simulink library "BrickPi"  (R2018b)
settings: Solver=VariableStepAuto  StartTime=0.0  StopTime=10.0  RelTol=1e-3
libraries: raspberrypilib x50, hdlsllib x27, xpcutilitieslib x18, $bdroot x1
(part 2 of 4)

== system BrickPi/EV3_Infrared/Get_sensor_value ==
  SensorPort : Inport
  SensorType : Inport  Port=2
  Enable : EnablePort
  Merge2 : Merge  Inputs=3
  Subsystem : Subsystem
  Subsystem1 : Subsystem
  Subsystem2 : Subsystem
  Switch Case : SwitchCase  CaseConditions={1,2,3}
  Terminator : Terminator
  Proximity : Outport
  Heading : Outport  Port=2
  Distance : Outport  Port=3
  Remote : Outport  Port=4
  Error : Outport  Port=5
  wires:
  SensorType/1 -> Subsystem2/2(SensorType), Subsystem1/2(SensorType), Subsystem/2(SensorType), Switch Case/1
  Switch Case/4 -> Terminator/1
  Switch Case/1 -> Subsystem/Action
  Subsystem/1(Proximity) -> Proximity/1
  Subsystem/2(Error) -> Merge2/1
  Subsystem1/3(Error) -> Merge2/2
  Switch Case/2 -> Subsystem1/Action
  Merge2/1 -> Error/1
  Subsystem2/2(Error) -> Merge2/3
  Switch Case/3 -> Subsystem2/Action
  Subsystem1/1(Heading) -> Heading/1
  Subsystem1/2(Distance) -> Distance/1
  Subsystem2/1(Remote) -> Remote/1
  SensorPort/1 -> Subsystem/1(SensorPort), Subsystem1/1(SensorPort), Subsystem2/1(SensorPort)

== system BrickPi/EV3_Infrared/Set_sensor_type ==
  note: Check whether 4th element == 0xA5?
  note: Set sensor type
  SensorPort : Inport  OutDataTypeStr=uint8
  SensorType : Inport  Port=2
  Enable : EnablePort
  0xA5 : Constant  Value=165
  Add : Sum
  Address : Constant  VectorParams1D=off  OutDataTypeStr=uint8
  Constant2 : Constant  OutDataTypeStr=uint8
  Constant3 : Constant  OutDataTypeStr=uint8
  Mux1 : Mux
  NAND : Logic  Operator=NAND  IconShape=distinctive  AllPortsSameDT=off  OutDataTypeStr=boolean
  SPI Master Transfer1 : raspberrypilib/SPI Master Transfer  Priority=1  BoardProperty=Pi 3 Model B  SPIModule=uint32(0)  Mode=Master  BusSpeed=1000000  Pin=SPI0_CE1  FirstBitToTransfer=Most significant bit (MSB)  ClockMode=0  BlockFunction=Transfer  RegisterAddress=0  OutputDataType=int8  OutputDataLength=1
      settings: SourceProductName=Simulink Support Package for Raspberry Pi Hardware  SourceProductBaseCode=RASPPI
  SPI_MSG_SET_ SENSOR_TYPE : Constant  Value=12  OutMin=[1]  OutMax=[28]  OutDataTypeStr=uint8
  Selector1 : Selector  InputPortWidth=4  IndexOptions=Index vector (dialog)  Indices=[4]  OutputSizes=1
  Shift Arithmetic : ArithShift  BitShiftNumberSource=Input port  BitShiftNumber=8  BitShiftDirection=Left
      settings: InputPortMap=u0,p1
  Subtract : Sum  Inputs=+-
  Type Offset : Constant  Value=25  OutDataTypeStr=uint8
  Error : Outport
  wires:
  Mux1/1 -> SPI Master Transfer1/1
  SPI Master Transfer1/1 -> Selector1/1
  Address/1 -> Mux1/1
  SPI_MSG_SET_ SENSOR_TYPE/1 -> Mux1/2
  Selector1/1 -> NAND/1
  0xA5/1 -> NAND/2
  NAND/1 -> Error/1
  Subtract/1 -> Shift Arithmetic/2
  Constant3/1 -> Subtract/2
  SensorPort/1 -> Subtract/1
  Constant2/1 -> Shift Arithmetic/1
  Shift Arithmetic/1 -> Mux1/3
  SensorType/1 -> Add/1
  Type Offset/1 -> Add/2
  Add/1 -> Mux1/4

== system BrickPi/EV3_Ultrasonic/Get_sensor_value ==
  note: Which sensor type has been selected?
  SensorPort : Inport
  SensorType : Inport  Port=2  OutDataTypeStr=uint8
  Enable : EnablePort
  CM_INCHES : Subsystem
  LISTEN : Subsystem
  Merge1 : Merge
  Switch Case : SwitchCase  CaseConditions={[1,2],3}
  Terminator : Terminator
  cm : Outport
  inch : Outport  Port=2
  pres : Outport  Port=3
  Error : Outport  Port=4
  wires:
  SensorType/1 -> CM_INCHES/2(SensorType), Switch Case/1
  Switch Case/1 -> CM_INCHES/Action
  Switch Case/2 -> LISTEN/Action
  SensorPort/1 -> CM_INCHES/1(SensorPort), LISTEN/1(SensorPort)
  CM_INCHES/1(cm) -> cm/1
  Merge1/1 -> Error/1
  CM_INCHES/3(Error) -> Merge1/1
  LISTEN/2(Error) -> Merge1/2
  LISTEN/1(presence) -> pres/1
  CM_INCHES/2(inch) -> inch/1
  Switch Case/3 -> Terminator/1

== system BrickPi/EV3_Ultrasonic/Set_sensor_type ==
  note: Set sensor type
  note: Check whether 4th element == 0xA5?
  SensorPort : Inport  OutDataTypeStr=uint8
  SensorType : Inport  Port=2  OutDataTypeStr=uint8
  Enable : EnablePort
  0xA5 : Constant  Value=165
  Address : Constant  VectorParams1D=off  OutDataTypeStr=uint8
  Constant2 : Constant  OutDataTypeStr=uint8
  Constant3 : Constant  OutDataTypeStr=uint8
  Mux1 : Mux
  NAND : Logic  Operator=NAND  IconShape=distinctive  AllPortsSameDT=off  OutDataTypeStr=boolean
  SPI Master Transfer1 : raspberrypilib/SPI Master Transfer  Priority=1  BoardProperty=Pi 3 Model B  SPIModule=uint32(0)  Mode=Master  BusSpeed=1000000  Pin=SPI0_CE1  FirstBitToTransfer=Most significant bit (MSB)  ClockMode=0  BlockFunction=Transfer  RegisterAddress=0  OutputDataType=int8  OutputDataLength=1
      settings: SourceProductName=Simulink Support Package for Raspberry Pi Hardware  SourceProductBaseCode=RASPPI
  SPI_MSG_SET_ SENSOR_TYPE : Constant  Value=12  OutMin=[1]  OutMax=[28]  OutDataTypeStr=uint8
  Selector1 : Selector  InputPortWidth=4  IndexOptions=Index vector (dialog)  Indices=[4]  OutputSizes=1
  Sensor type offset : Constant  Value=22  OutDataTypeStr=uint8
  Shift Arithmetic : ArithShift  BitShiftNumberSource=Input port  BitShiftNumber=8  BitShiftDirection=Left
      settings: InputPortMap=u0,p1
  Subtract : Sum  Inputs=+-
  Sum : Sum
  Error : Outport  InitialOutput=[1]
  wires:
  Sensor type offset/1 -> Sum/2
  SensorType/1 -> Sum/1
  Sum/1 -> Mux1/4
  Shift Arithmetic/1 -> Mux1/3
  Constant2/1 -> Shift Arithmetic/1
  SensorPort/1 -> Subtract/1
  Constant3/1 -> Subtract/2
  Subtract/1 -> Shift Arithmetic/2
  NAND/1 -> Error/1
  0xA5/1 -> NAND/2
  Selector1/1 -> NAND/1
  SPI_MSG_SET_ SENSOR_TYPE/1 -> Mux1/2
  Address/1 -> Mux1/1
  SPI Master Transfer1/1 -> Selector1/1
  Mux1/1 -> SPI Master Transfer1/1

== system BrickPi/Motor_Encoder/Get Encoder Value ==
  note: Use only when "Reset on external signal" selected
  note: Get motor encoder
  MotorPort : Inport
  ResetMode : Inport  Port=2
  ExtSignal : Inport  Port=3
  Enable : EnablePort
  0xA5 : Constant  Value=165
  "Address " : Constant  OutDataTypeStr=uint8
  Address3 : Constant  Value=[0 0 0 0 0 0 0 0]  OutDataTypeStr=uint8
  "Byte Packing " : xpcutilitieslib/Byte Packing   MaskPackedDataType=int32  MaskUnpackedDataTypes={'uint8', 'uint8', 'uint8', 'uint8'}  MaskAlignment=1
  Bytes[3-7] : Selector  IndexMode=Zero-based  InputPortWidth=10  IndexOptions=Index vector (dialog)  Indices=[3 4 5 6 7]  OutputSizes=1
  Demux : Demux  Outputs=5
  Mux2 : Mux  Inputs=3
  NAND : Logic  Operator=NAND  IconShape=distinctive  AllPortsSameDT=off  OutDataTypeStr=boolean
  SPI Master Transfer2 : raspberrypilib/SPI Master Transfer  Priority=6  BoardProperty=Pi 3 Model B  SPIModule=uint32(0)  Mode=Master  BusSpeed=1000000  Pin=SPI0_CE1  FirstBitToTransfer=Most significant bit (MSB)  ClockMode=0  BlockFunction=Transfer  RegisterAddress=0  OutputDataType=int8  OutputDataLength=1
      settings: SourceProductName=Simulink Support Package for Raspberry Pi Hardware  SourceProductBaseCode=RASPPI
  SPI_MSG_GET_ MOTOR_ENCODER offset : Constant  Value=29  OutDataTypeStr=uint8
  Sum : Sum  OutDataTypeStr=uint8
  Switch Case : SwitchCase
  Switch Case Action Subsystem : Subsystem  TreatAsAtomicUnit=on
  Terminator : Terminator
  Value : Outport
  Error : Outport  Port=2
  wires:
  SPI_MSG_GET_ MOTOR_ENCODER offset/1 -> Sum/2
  SPI Master Transfer2/1 -> Bytes[3-7]/1
  Bytes[3-7]/1 -> Demux/1
  "Byte Packing "/1 -> Value/1
  Demux/2 -> "Byte Packing "/4
  0xA5/1 -> NAND/1
  Demux/1 -> NAND/2
  Demux/3 -> "Byte Packing "/3
  Demux/4 -> "Byte Packing "/2
  "Address "/1 -> Mux2/1
  Demux/5 -> "Byte Packing "/1
  MotorPort/1 -> Switch Case Action Subsystem/2(MotorPort), Sum/1
  Mux2/1 -> SPI Master Transfer2/1
  Sum/1 -> Mux2/2
  NAND/1 -> Error/1
  Address3/1 -> Mux2/3
  ResetMode/1 -> Switch Case/1
  Switch Case/2 -> Terminator/1
  Switch Case/1 -> Switch Case Action Subsystem/Action
  ExtSignal/1 -> Switch Case Action Subsystem/1(ExtSignal)

== system BrickPi/Motor_Encoder/Reset Encoder once ==
  MotorPort : Inport
  Enable : EnablePort
  Encoder : Subsystem  AncestorBlock=BrickPi/Motor_Encoder/Subsystem
  Motor_Offset : Subsystem
  Error : Outport
  wires:
  Encoder/1(Value) -> Motor_Offset/1(Offset)
  MotorPort/1 -> Motor_Offset/2(MotorPort), Encoder/1(MotorPort)
  Encoder/2(Error) -> Error/1

== system BrickPi/Motor_Offset/If Action Subsystem ==
  note: Set offset value
  Offset : Inport
  Action Port : ActionPort  ActionType=then
  "Address " : Constant  OutDataTypeStr=uint8
  Bit Shift : hdlsllib/Logic and Bit Operations/Bit Shift  mode=Shift Right Logical  N=24
      settings: SourceProductName=HDL Coder  SourceProductBaseCode=HD
  Bit Shift1 : hdlsllib/Logic and Bit Operations/Bit Shift  mode=Shift Right Logical  N=16
      settings: SourceProductName=HDL Coder  SourceProductBaseCode=HD
  Bit Shift2 : hdlsllib/Logic and Bit Operations/Bit Shift  mode=Shift Right Logical  N=8
      settings: SourceProductName=HDL Coder  SourceProductBaseCode=HD
  "Byte Unpacking " : xpcutilitieslib/Byte Unpacking   MaskUnpackedDataTypes={'uint8'}  MaskUnpackedDataSizes={[1]}  MaskAlignment=1
      settings: SourceProductName=Simulink Real-Time  SourceProductBaseCode=XP
  Constant2 : Constant  OutDataTypeStr=uint8
  Constant3 : Constant  OutDataTypeStr=uint8
  Data Type Conversion{,1..3} (4 alike) : DataTypeConversion  OutDataTypeStr=uint8
  MotorPort : Constant  Value=MotorPort  OutDataTypeStr=uint8
  Mux2 : Mux  Inputs=7
  SPI Master Transfer2 : raspberrypilib/SPI Master Transfer  Priority=6  BoardProperty=Pi 3 Model B  SPIModule=uint32(0)  Mode=Master  BusSpeed=1000000  Pin=SPI0_CE1  FirstBitToTransfer=Most significant bit (MSB)  ClockMode=0  BlockFunction=Transfer  RegisterAddress=0  OutputDataType=int8  OutputDataLength=1
      settings: SourceProductName=Simulink Support Package for Raspberry Pi Hardware  SourceProductBaseCode=RASPPI
  SPI_MSG_ OFFSET_ENCODER : Constant  Value=29  OutMin=[1]  OutDataTypeStr=uint8
  Shift Arithmetic : ArithShift  BitShiftNumberSource=Input port  BitShiftNumber=8  BitShiftDirection=Left
      settings: InputPortMap=u0,p1
  Subtract : Sum  Inputs=+-
  Terminator : Terminator
  wires:
  Data Type Conversion2/1 -> Mux2/6
  Constant2/1 -> Shift Arithmetic/1
  Data Type Conversion/1 -> Mux2/4
  Data Type Conversion3/1 -> Mux2/7
  MotorPort/1 -> Subtract/1
  SPI_MSG_ OFFSET_ENCODER/1 -> Mux2/2
  Subtract/1 -> Shift Arithmetic/2
  SPI Master Transfer2/1 -> Terminator/1
  Data Type Conversion1/1 -> Mux2/5
  "Address "/1 -> Mux2/1
  Bit Shift1/1 -> Data Type Conversion1/1
  Constant3/1 -> Subtract/2
  Bit Shift/1 -> Data Type Conversion/1
  Mux2/1 -> SPI Master Transfer2/1
  Shift Arithmetic/1 -> Mux2/3
  Bit Shift2/1 -> Data Type Conversion2/1
  Offset/1 -> Bit Shift1/1, Bit Shift2/1, Data Type Conversion3/1, Bit Shift/1

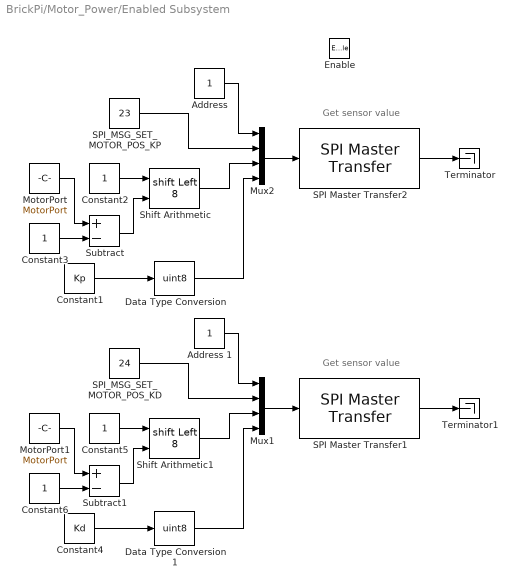
== system BrickPi/Motor_Power/Enabled Subsystem ==
  note: Get sensor value
  note: Get sensor value
  Enable : EnablePort
  "Address " : Constant  OutDataTypeStr=uint8
  Address 1 : Constant  OutDataTypeStr=uint8
  Constant1 : Constant  Value=Kp
  Constant{2..3,5..6} (4 alike) : Constant  OutDataTypeStr=uint8
  Constant4 : Constant  Value=Kd
  Data Type Conversion : DataTypeConversion  OutDataTypeStr=uint8
  Data Type Conversion1 : DataTypeConversion  OutDataTypeStr=uint8
  MotorPort : Constant  Value=MotorPort  OutDataTypeStr=uint8
  MotorPort1 : Constant  Value=MotorPort  OutDataTypeStr=uint8
  Mux1 : Mux
  Mux2 : Mux
  SPI Master Transfer1 : raspberrypilib/SPI Master Transfer  Priority=6  BoardProperty=Pi 3 Model B  SPIModule=uint32(0)  Mode=Master  BusSpeed=1000000  Pin=SPI0_CE1  FirstBitToTransfer=Most significant bit (MSB)  ClockMode=0  BlockFunction=Transfer  RegisterAddress=0  OutputDataType=int8  OutputDataLength=1
      settings: SourceProductName=Simulink Support Package for Raspberry Pi Hardware  SourceProductBaseCode=RASPPI
  SPI Master Transfer2 : raspberrypilib/SPI Master Transfer  Priority=6  BoardProperty=Pi 3 Model B  SPIModule=uint32(0)  Mode=Master  BusSpeed=1000000  Pin=SPI0_CE1  FirstBitToTransfer=Most significant bit (MSB)  ClockMode=0  BlockFunction=Transfer  RegisterAddress=0  OutputDataType=int8  OutputDataLength=1
      settings: SourceProductName=Simulink Support Package for Raspberry Pi Hardware  SourceProductBaseCode=RASPPI
  SPI_MSG_SET_ MOTOR_POS_KD : Constant  Value=24  OutMin=[1]  OutMax=[28]  OutDataTypeStr=uint8
  SPI_MSG_SET_ MOTOR_POS_KP : Constant  Value=23  OutMin=[1]  OutMax=[28]  OutDataTypeStr=uint8
  Shift Arithmetic : ArithShift  BitShiftNumberSource=Input port  BitShiftNumber=8  BitShiftDirection=Left
      settings: InputPortMap=u0,p1
  Shift Arithmetic1 : ArithShift  BitShiftNumberSource=Input port  BitShiftNumber=8  BitShiftDirection=Left
      settings: InputPortMap=u0,p1
  Subtract : Sum  Inputs=+-
  Subtract1 : Sum  Inputs=+-
  Terminator : Terminator
  Terminator1 : Terminator
  wires:
  SPI_MSG_SET_ MOTOR_POS_KP/1 -> Mux2/2
  Constant3/1 -> Subtract/2
  SPI Master Transfer2/1 -> Terminator/1
  Constant1/1 -> Data Type Conversion/1
  Data Type Conversion/1 -> Mux2/4
  MotorPort/1 -> Subtract/1
  Shift Arithmetic/1 -> Mux2/3
  "Address "/1 -> Mux2/1
  Constant2/1 -> Shift Arithmetic/1
  Mux2/1 -> SPI Master Transfer2/1
  Subtract/1 -> Shift Arithmetic/2
  Subtract1/1 -> Shift Arithmetic1/2
  Constant5/1 -> Shift Arithmetic1/1
  MotorPort1/1 -> Subtract1/1
  Mux1/1 -> SPI Master Transfer1/1
  Address 1/1 -> Mux1/1
  Shift Arithmetic1/1 -> Mux1/3
  Constant6/1 -> Subtract1/2
  Data Type Conversion1/1 -> Mux1/4
  SPI Master Transfer1/1 -> Terminator1/1
  SPI_MSG_SET_ MOTOR_POS_KD/1 -> Mux1/2
  Constant4/1 -> Data Type Conversion1/1

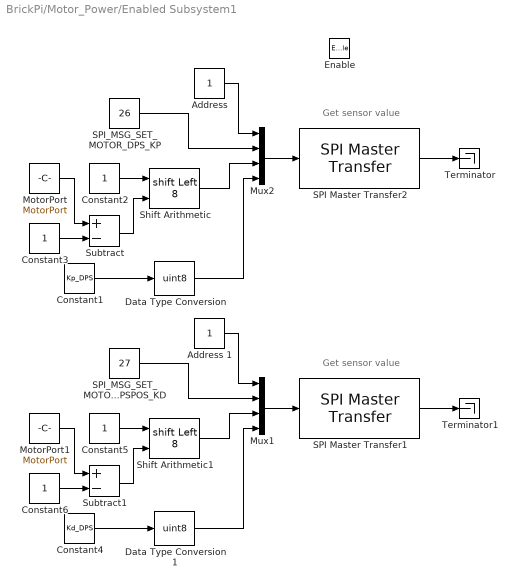
== system BrickPi/Motor_Power/Enabled Subsystem1 ==
  note: Get sensor value
  note: Get sensor value
  Enable : EnablePort
  "Address " : Constant  OutDataTypeStr=uint8
  Address 1 : Constant  OutDataTypeStr=uint8
  Constant1 : Constant  Value=Kp_DPS
  Constant{2..3,5..6} (4 alike) : Constant  OutDataTypeStr=uint8
  Constant4 : Constant  Value=Kd_DPS
  Data Type Conversion : DataTypeConversion  OutDataTypeStr=uint8
  Data Type Conversion1 : DataTypeConversion  OutDataTypeStr=uint8
  MotorPort : Constant  Value=MotorPort  OutDataTypeStr=uint8
  MotorPort1 : Constant  Value=MotorPort  OutDataTypeStr=uint8
  Mux1 : Mux
  Mux2 : Mux
  SPI Master Transfer1 : raspberrypilib/SPI Master Transfer  Priority=6  BoardProperty=Pi 3 Model B  SPIModule=uint32(0)  Mode=Master  BusSpeed=1000000  Pin=SPI0_CE1  FirstBitToTransfer=Most significant bit (MSB)  ClockMode=0  BlockFunction=Transfer  RegisterAddress=0  OutputDataType=int8  OutputDataLength=1
      settings: SourceProductName=Simulink Support Package for Raspberry Pi Hardware  SourceProductBaseCode=RASPPI
  SPI Master Transfer2 : raspberrypilib/SPI Master Transfer  Priority=6  BoardProperty=Pi 3 Model B  SPIModule=uint32(0)  Mode=Master  BusSpeed=1000000  Pin=SPI0_CE1  FirstBitToTransfer=Most significant bit (MSB)  ClockMode=0  BlockFunction=Transfer  RegisterAddress=0  OutputDataType=int8  OutputDataLength=1
      settings: SourceProductName=Simulink Support Package for Raspberry Pi Hardware  SourceProductBaseCode=RASPPI
  SPI_MSG_SET_ MOTOR_DPSPOS_KD : Constant  Value=27  OutMin=[1]  OutMax=[28]  OutDataTypeStr=uint8
  SPI_MSG_SET_ MOTOR_DPS_KP : Constant  Value=26  OutMin=[1]  OutMax=[28]  OutDataTypeStr=uint8
  Shift Arithmetic : ArithShift  BitShiftNumberSource=Input port  BitShiftNumber=8  BitShiftDirection=Left
      settings: InputPortMap=u0,p1
  Shift Arithmetic1 : ArithShift  BitShiftNumberSource=Input port  BitShiftNumber=8  BitShiftDirection=Left
      settings: InputPortMap=u0,p1
  Subtract : Sum  Inputs=+-
  Subtract1 : Sum  Inputs=+-
  Terminator : Terminator
  Terminator1 : Terminator
  wires:
  SPI_MSG_SET_ MOTOR_DPS_KP/1 -> Mux2/2
  Constant3/1 -> Subtract/2
  SPI Master Transfer2/1 -> Terminator/1
  Constant1/1 -> Data Type Conversion/1
  Data Type Conversion/1 -> Mux2/4
  MotorPort/1 -> Subtract/1
  Shift Arithmetic/1 -> Mux2/3
  "Address "/1 -> Mux2/1
  Constant2/1 -> Shift Arithmetic/1
  Mux2/1 -> SPI Master Transfer2/1
  Subtract/1 -> Shift Arithmetic/2
  Subtract1/1 -> Shift Arithmetic1/2
  Constant5/1 -> Shift Arithmetic1/1
  MotorPort1/1 -> Subtract1/1
  Mux1/1 -> SPI Master Transfer1/1
  Address 1/1 -> Mux1/1
  Shift Arithmetic1/1 -> Mux1/3
  Constant6/1 -> Subtract1/2
  Data Type Conversion1/1 -> Mux1/4
  SPI Master Transfer1/1 -> Terminator1/1
  SPI_MSG_SET_ MOTOR_DPSPOS_KD/1 -> Mux1/2
  Constant4/1 -> Data Type Conversion1/1

== system BrickPi/Motor_Power/Subsystem ==
  Choice : Inport
  Power : Inport  Port=2
  Position : Inport  Port=3
  DPS : Inport  Port=4
  Action Port : ActionPort  ActionType=then
  Set_DPS : Subsystem
  Set_Limit : Subsystem
  Set_Position : Subsystem
  Set_Power : Subsystem
  Switch Case : SwitchCase  CaseConditions={1,2,3,4}
  Terminator : Terminator
  wires:
  Switch Case/3 -> Set_DPS/Action
  DPS/1 -> Set_DPS/1(DPS), Set_Limit/2(DPS)
  Switch Case/1 -> Set_Power/Action
  Power/1 -> Set_Power/1(Power), Set_Limit/1(Power)
  Choice/1 -> Switch Case/1
  Switch Case/5 -> Terminator/1
  Position/1 -> Set_Position/1(Position)
  Switch Case/2 -> Set_Position/Action
  Switch Case/4 -> Set_Limit/Action

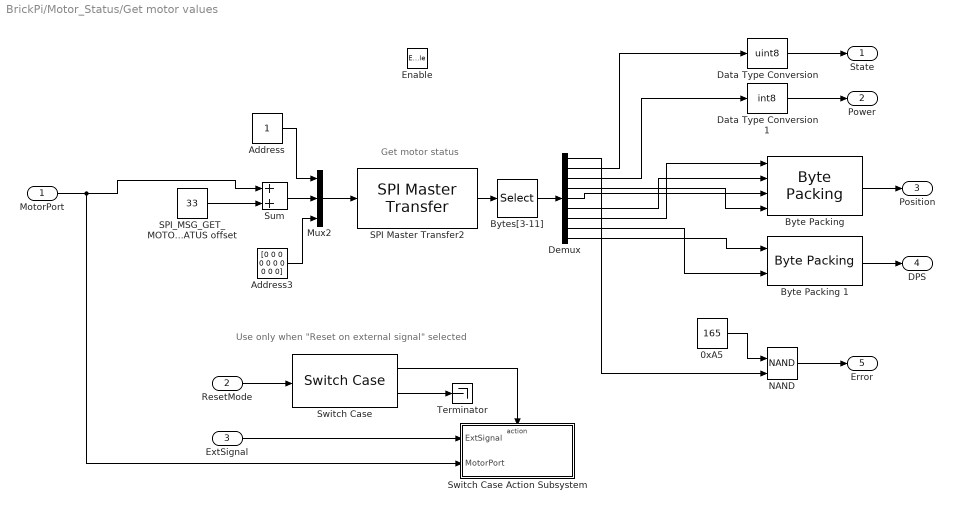
== system BrickPi/Motor_Status/Get motor values ==
  note: Get motor status
  note: Use only when "Reset on external signal" selected
  MotorPort : Inport
  ResetMode : Inport  Port=2
  ExtSignal : Inport  Port=3
  Enable : EnablePort
  0xA5 : Constant  Value=165
  "Address " : Constant  OutDataTypeStr=uint8
  Address3 : Constant  Value=[0 0 0 0 0 0 0 0 0 0]  OutDataTypeStr=uint8
  "Byte Packing " : xpcutilitieslib/Byte Packing   MaskPackedDataType=int32  MaskUnpackedDataTypes={'uint8', 'uint8', 'uint8', 'uint8'}  MaskAlignment=1
  Byte Packing 1 : xpcutilitieslib/Byte Packing   MaskPackedDataType=int16  MaskUnpackedDataTypes={'uint8','uint8'}  MaskAlignment=1
  Bytes[3-11] : Selector  IndexMode=Zero-based  InputPortWidth=12  IndexOptions=Index vector (dialog)  Indices=[3 4 5 6 7 8 9 10 11]  OutputSizes=1
  Data Type Conversion : DataTypeConversion  OutDataTypeStr=uint8
  Data Type Conversion1 : DataTypeConversion  OutDataTypeStr=int8
  Demux : Demux  Outputs=9
  Mux2 : Mux  Inputs=3
  NAND : Logic  Operator=NAND  IconShape=distinctive  AllPortsSameDT=off  OutDataTypeStr=boolean
  SPI Master Transfer2 : raspberrypilib/SPI Master Transfer  Priority=6  BoardProperty=Pi 3 Model B  SPIModule=uint32(0)  Mode=Master  BusSpeed=1000000  Pin=SPI0_CE1  FirstBitToTransfer=Most significant bit (MSB)  ClockMode=0  BlockFunction=Transfer  RegisterAddress=0  OutputDataType=int8  OutputDataLength=1
      settings: SourceProductName=Simulink Support Package for Raspberry Pi Hardware  SourceProductBaseCode=RASPPI
  SPI_MSG_GET_ MOTOR_STATUS offset : Constant  Value=33  OutMin=[1]  OutDataTypeStr=uint8
  Sum : Sum  OutDataTypeStr=uint8
  Switch Case : SwitchCase
  Switch Case Action Subsystem : Subsystem  TreatAsAtomicUnit=on
  Terminator : Terminator
  State : Outport
  Power : Outport  Port=2
  Position : Outport  Port=3
  DPS : Outport  Port=4
  Error : Outport  Port=5
  wires:
  Demux/2 -> Data Type Conversion/1
  Mux2/1 -> SPI Master Transfer2/1
  "Address "/1 -> Mux2/1
  Demux/9 -> Byte Packing 1/1
  Demux/1 -> NAND/2
  Demux/7 -> "Byte Packing "/1
  Demux/6 -> "Byte Packing "/2
  Bytes[3-11]/1 -> Demux/1
  SPI Master Transfer2/1 -> Bytes[3-11]/1
  Demux/8 -> Byte Packing 1/2
  SPI_MSG_GET_ MOTOR_STATUS offset/1 -> Sum/2
  Sum/1 -> Mux2/2
  MotorPort/1 -> Switch Case Action Subsystem/2(MotorPort), Sum/1
  0xA5/1 -> NAND/1
  Demux/3 -> Data Type Conversion1/1
  Address3/1 -> Mux2/3
  Demux/5 -> "Byte Packing "/3
  Demux/4 -> "Byte Packing "/4
  Byte Packing 1/1 -> DPS/1
  "Byte Packing "/1 -> Position/1
  NAND/1 -> Error/1
  Data Type Conversion1/1 -> Power/1
  Data Type Conversion/1 -> State/1
  ExtSignal/1 -> Switch Case Action Subsystem/1(ExtSignal)
  ResetMode/1 -> Switch Case/1
  Switch Case/1 -> Switch Case Action Subsystem/Action
  Switch Case/2 -> Terminator/1

== system BrickPi/Motor_Status/Reset Encoder once ==
  MotorPort : Inport
  Enable : EnablePort
  Encoder : Subsystem  AncestorBlock=BrickPi/Motor_Encoder/Subsystem
  Motor_Offset : Subsystem
  Error : Outport
  wires:
  Encoder/1(Value) -> Motor_Offset/1(Offset)
  MotorPort/1 -> Motor_Offset/2(MotorPort), Encoder/1(MotorPort)
  Encoder/2(Error) -> Error/1

== system BrickPi/NXT_Color/Get_sensor_value ==
  note: Which sensor type has been selected?
  SensorPort : Inport
  SensorType : Inport  Port=2  OutDataTypeStr=uint8
  Enable : EnablePort
  FULL : Subsystem
  Merge : Merge
  Merge1 : Merge
  R_G_B_OFF : Subsystem
  Switch Case : SwitchCase  CaseConditions={[1,2,3,5],4}
  Terminator : Terminator
  Values : Outport
  Error : Outport  Port=2
  wires:
  Switch Case/1 -> R_G_B_OFF/Action
  SensorType/1 -> R_G_B_OFF/2(SensorType), Switch Case/1
  Switch Case/2 -> FULL/Action
  SensorPort/1 -> R_G_B_OFF/1(SensorPort), FULL/1(SensorPort)
  Merge/1 -> Error/1
  FULL/2(Error) -> Merge/2
  R_G_B_OFF/2(Error) -> Merge/1
  Merge1/1 -> Values/1
  R_G_B_OFF/1(Value) -> Merge1/1
  FULL/1(Value) -> Merge1/2
  Switch Case/3 -> Terminator/1

== system BrickPi/NXT_Color/Set_sensor_type ==
  note: Set sensor type
  note: Check whether 4th element == 0xA5?
  SensorPort : Inport  OutDataTypeStr=uint8
  SensorType : Inport  Port=2  OutDataTypeStr=uint8
  Enable : EnablePort
  0xA5 : Constant  Value=165
  Address : Constant  VectorParams1D=off  OutDataTypeStr=uint8
  Constant2 : Constant  OutDataTypeStr=uint8
  Constant3 : Constant  OutDataTypeStr=uint8
  Mux1 : Mux
  NAND : Logic  Operator=NAND  IconShape=distinctive  AllPortsSameDT=off  OutDataTypeStr=boolean
  SPI Master Transfer1 : raspberrypilib/SPI Master Transfer  Priority=1  BoardProperty=Pi 3 Model B  SPIModule=uint32(0)  Mode=Master  BusSpeed=1000000  Pin=SPI0_CE1  FirstBitToTransfer=Most significant bit (MSB)  ClockMode=0  BlockFunction=Transfer  RegisterAddress=0  OutputDataType=int8  OutputDataLength=1
      settings: SourceProductName=Simulink Support Package for Raspberry Pi Hardware  SourceProductBaseCode=RASPPI
  SPI_MSG_SET_ SENSOR_TYPE : Constant  Value=12  OutMin=[1]  OutMax=[28]  OutDataTypeStr=uint8
  Selector1 : Selector  InputPortWidth=4  IndexOptions=Index vector (dialog)  Indices=[4]  OutputSizes=1
  Sensor type offset : Constant  Value=8  OutDataTypeStr=uint8
  Shift Arithmetic : ArithShift  BitShiftNumberSource=Input port  BitShiftNumber=8  BitShiftDirection=Left
      settings: InputPortMap=u0,p1
  Subtract : Sum  Inputs=+-
  Sum : Sum
  Error : Outport
  wires:
  Sensor type offset/1 -> Sum/2
  SensorType/1 -> Sum/1
  Sum/1 -> Mux1/4
  Shift Arithmetic/1 -> Mux1/3
  Constant2/1 -> Shift Arithmetic/1
  SensorPort/1 -> Subtract/1
  Constant3/1 -> Subtract/2
  Subtract/1 -> Shift Arithmetic/2
  NAND/1 -> Error/1
  0xA5/1 -> NAND/2
  Selector1/1 -> NAND/1
  SPI_MSG_SET_ SENSOR_TYPE/1 -> Mux1/2
  Address/1 -> Mux1/1
  SPI Master Transfer1/1 -> Selector1/1
  Mux1/1 -> SPI Master Transfer1/1

== system BrickPi/NXT_Light/Get_sensor_value ==
  note: Get sensor value
  SensorPort : Inport
  SensorType : Inport  Port=2  OutDataTypeStr=uint8
  Enable : EnablePort
  0xA5 : Constant  Value=165
  "Address " : Constant  OutDataTypeStr=uint8
  Address3 : Constant  Value=[0 0 0 0 0 0]  OutDataTypeStr=uint8
  "Byte Packing " : xpcutilitieslib/Byte Packing   MaskPackedDataType=uint16  MaskUnpackedDataTypes={'uint8', 'uint8'}  MaskAlignment=1
  Bytes[3-7] : Selector  IndexMode=Zero-based  InputPortWidth=8  IndexOptions=Index vector (dialog)  Indices=[3 4 5 6 7]  OutputSizes=1
  Demux : Demux  Outputs=5
  Equal : RelationalOperator  Operator=~=  OutDataTypeStr=boolean  RndMeth=Simplest
  Equal1 : RelationalOperator  Operator=~=  OutDataTypeStr=boolean  RndMeth=Simplest
  Equal2 : RelationalOperator  Operator=~=  OutDataTypeStr=boolean  RndMeth=Simplest
  Mux : Mux  Inputs=3
  Mux2 : Mux  Inputs=3
  SPI Master Transfer2 : raspberrypilib/SPI Master Transfer  Priority=6  BoardProperty=Pi 3 Model B  SPIModule=uint32(0)  Mode=Master  BusSpeed=1000000  Pin=SPI0_CE1  FirstBitToTransfer=Most significant bit (MSB)  ClockMode=0  BlockFunction=Transfer  RegisterAddress=0  OutputDataType=int8  OutputDataLength=1
      settings: SourceProductName=Simulink Support Package for Raspberry Pi Hardware  SourceProductBaseCode=RASPPI
  SPI_MSG_GET_ SENSOR offset : Constant  Value=12  OutMin=[1]  OutMax=[28]  OutDataTypeStr=uint8
  Sensor type offset : Constant  Value=6  OutDataTypeStr=uint8
  Sum : Sum  OutDataTypeStr=uint8
  Sum1 : Sum
  Valid data : Constant  Value=0  OutDataTypeStr=uint8
  Value : Outport
  Error : Outport  Port=2
  wires:
  Sensor type offset/1 -> Sum1/2
  SensorType/1 -> Sum1/1
  Sum1/1 -> Equal/1
  Equal2/1 -> Mux/1
  Demux/1 -> Equal2/2
  Equal1/1 -> Mux/3
  Mux/1 -> Error/1
  Equal/1 -> Mux/2
  Demux/3 -> Equal1/1
  Valid data/1 -> Equal1/2
  0xA5/1 -> Equal2/1
  Demux/2 -> Equal/2
  Bytes[3-7]/1 -> Demux/1
  SensorPort/1 -> Sum/1
  SPI_MSG_GET_ SENSOR offset/1 -> Sum/2
  Sum/1 -> Mux2/2
  "Address "/1 -> Mux2/1
  Mux2/1 -> SPI Master Transfer2/1
  SPI Master Transfer2/1 -> Bytes[3-7]/1
  Address3/1 -> Mux2/3
  "Byte Packing "/1 -> Value/1
  Demux/4 -> "Byte Packing "/2
  Demux/5 -> "Byte Packing "/1

== system BrickPi/NXT_Light/Set_sensor_type ==
  note: Set sensor type
  note: Check whether 4th element == 0xA5?
  SensorPort : Inport  OutDataTypeStr=uint8
  SensorType : Inport  Port=2  OutDataTypeStr=uint8
  Enable : EnablePort
  0xA5 : Constant  Value=165
  Address : Constant  VectorParams1D=off  OutDataTypeStr=uint8
  Constant2 : Constant  OutDataTypeStr=uint8
  Constant3 : Constant  OutDataTypeStr=uint8
  Mux1 : Mux
  NAND : Logic  Operator=NAND  IconShape=distinctive  AllPortsSameDT=off  OutDataTypeStr=boolean
  SPI Master Transfer1 : raspberrypilib/SPI Master Transfer  Priority=1  BoardProperty=Pi 3 Model B  SPIModule=uint32(0)  Mode=Master  BusSpeed=1000000  Pin=SPI0_CE1  FirstBitToTransfer=Most significant bit (MSB)  ClockMode=0  BlockFunction=Transfer  RegisterAddress=0  OutputDataType=int8  OutputDataLength=1
      settings: SourceProductName=Simulink Support Package for Raspberry Pi Hardware  SourceProductBaseCode=RASPPI
  SPI_MSG_SET_ SENSOR_TYPE : Constant  Value=12  OutMin=[1]  OutMax=[28]  OutDataTypeStr=uint8
  Selector1 : Selector  InputPortWidth=4  IndexOptions=Index vector (dialog)  Indices=[4]  OutputSizes=1
  Sensor type offset : Constant  Value=6  OutDataTypeStr=uint8
  Shift Arithmetic : ArithShift  BitShiftNumberSource=Input port  BitShiftNumber=8  BitShiftDirection=Left
      settings: InputPortMap=u0,p1
  Subtract : Sum  Inputs=+-
  Sum : Sum
  Error : Outport
  wires:
  Sensor type offset/1 -> Sum/2
  SensorType/1 -> Sum/1
  Sum/1 -> Mux1/4
  Shift Arithmetic/1 -> Mux1/3
  Constant2/1 -> Shift Arithmetic/1
  SensorPort/1 -> Subtract/1
  Constant3/1 -> Subtract/2
  Subtract/1 -> Shift Arithmetic/2
  NAND/1 -> Error/1
  0xA5/1 -> NAND/2
  Selector1/1 -> NAND/1
  SPI_MSG_SET_ SENSOR_TYPE/1 -> Mux1/2
  Address/1 -> Mux1/1
  SPI Master Transfer1/1 -> Selector1/1
  Mux1/1 -> SPI Master Transfer1/1

== system BrickPi/NXT_Ultrasonic/Get_sensor_value ==
  note: Get sensor value
  SensorPort : Inport
  Enable : EnablePort
  0xA5 : Constant  Value=165
  "Address " : Constant  OutDataTypeStr=uint8
  Address3 : Constant  Value=[0 0 0 0 0]  OutDataTypeStr=uint8
  Bytes[3-6] : Selector  IndexMode=Zero-based  InputPortWidth=7  IndexOptions=Index vector (dialog)  Indices=[3 4 5 6]  OutputSizes=1
  Demux : Demux
  Mux : Mux  Inputs=3
  Mux2 : Mux  Inputs=3
  NAND : Logic  Operator=NAND  IconShape=distinctive  AllPortsSameDT=off  OutDataTypeStr=boolean
  NAND1 : Logic  Operator=NAND  IconShape=distinctive  AllPortsSameDT=off  OutDataTypeStr=boolean
  OR1 : Logic  Operator=OR  IconShape=distinctive  AllPortsSameDT=off  OutDataTypeStr=boolean
  SPI Master Transfer2 : raspberrypilib/SPI Master Transfer  Priority=6  BoardProperty=Pi 3 Model B  SPIModule=uint32(0)  Mode=Master  BusSpeed=1000000  Pin=SPI0_CE1  FirstBitToTransfer=Most significant bit (MSB)  ClockMode=0  BlockFunction=Transfer  RegisterAddress=0  OutputDataType=int8  OutputDataLength=1
      settings: SourceProductName=Simulink Support Package for Raspberry Pi Hardware  SourceProductBaseCode=RASPPI
  SPI_MSG_GET_ SENSOR offset : Constant  Value=12  OutMin=[1]  OutMax=[28]  OutDataTypeStr=uint8
  SensorType : Constant  Value=14  OutMin=[1]  OutMax=[28]  OutDataTypeStr=uint8
  Sum : Sum  OutDataTypeStr=uint8
  Valid data : Constant  Value=0  OutDataTypeStr=uint8
  Value : Outport
  Error : Outport  Port=2
  wires:
  Address3/1 -> Mux2/3
  SPI Master Transfer2/1 -> Bytes[3-6]/1
  Mux2/1 -> SPI Master Transfer2/1
  "Address "/1 -> Mux2/1
  Sum/1 -> Mux2/2
  SPI_MSG_GET_ SENSOR offset/1 -> Sum/2
  SensorPort/1 -> Sum/1
  Bytes[3-6]/1 -> Demux/1
  Demux/2 -> NAND1/2
  SensorType/1 -> NAND1/1
  Demux/4 -> Value/1
  0xA5/1 -> NAND/1
  Demux/1 -> NAND/2
  Valid data/1 -> OR1/2
  Demux/3 -> OR1/1
  NAND/1 -> Mux/1
  NAND1/1 -> Mux/2
  OR1/1 -> Mux/3
  Mux/1 -> Error/1

== system BrickPi/NXT_Ultrasonic/Set_sensor_type ==
  note: Check whether 4th element == 0xA5?
  note: Set sensor type
  SensorPort : Inport
  Enable : EnablePort
  0xA5 : Constant  Value=165
  Address : Constant  VectorParams1D=off  OutDataTypeStr=uint8
  Constant2 : Constant  OutDataTypeStr=uint8
  Constant3 : Constant  OutDataTypeStr=uint8
  Mux1 : Mux
  NAND : Logic  Operator=NAND  IconShape=distinctive  AllPortsSameDT=off  OutDataTypeStr=boolean
  SPI Master Transfer1 : raspberrypilib/SPI Master Transfer  Priority=1  BoardProperty=Pi 3 Model B  SPIModule=uint32(0)  Mode=Master  BusSpeed=1000000  Pin=SPI0_CE1  FirstBitToTransfer=Most significant bit (MSB)  ClockMode=0  BlockFunction=Transfer  RegisterAddress=0  OutputDataType=int8  OutputDataLength=1
      settings: SourceProductName=Simulink Support Package for Raspberry Pi Hardware  SourceProductBaseCode=RASPPI
  SPI_MSG_SET_ SENSOR_TYPE : Constant  Value=12  OutMin=[1]  OutMax=[28]  OutDataTypeStr=uint8
  Selector1 : Selector  InputPortWidth=4  IndexOptions=Index vector (dialog)  Indices=[4]  OutputSizes=1
  SensorType : Constant  Value=14  OutMin=[1]  OutMax=[28]  OutDataTypeStr=uint8
  Shift Arithmetic : ArithShift  BitShiftNumberSource=Input port  BitShiftNumber=8  BitShiftDirection=Left
      settings: InputPortMap=u0,p1
  Subtract : Sum  Inputs=+-
  Error : Outport  InitialOutput=[1]
  wires:
  Mux1/1 -> SPI Master Transfer1/1
  SPI Master Transfer1/1 -> Selector1/1
  Address/1 -> Mux1/1
  SPI_MSG_SET_ SENSOR_TYPE/1 -> Mux1/2
  SensorType/1 -> Mux1/4
  Selector1/1 -> NAND/1
  0xA5/1 -> NAND/2
  NAND/1 -> Error/1
  Subtract/1 -> Shift Arithmetic/2
  Constant3/1 -> Subtract/2
  SensorPort/1 -> Subtract/1
  Constant2/1 -> Shift Arithmetic/1
  Shift Arithmetic/1 -> Mux1/3

== system BrickPi/Reset_all/Reset motor power ==
  MOTOR_FLOAT : Constant  Value=-128  OutDataTypeStr=int8
  OR : Logic  Operator=OR  Inputs=4  IconShape=distinctive  AllPortsSameDT=off  OutDataTypeStr=boolean
  Reset power 1 : Subsystem
  Reset power 2 : Subsystem
  Reset power 3 : Subsystem
  Reset power 4 : Subsystem
  Error : Outport
  wires:
  MOTOR_FLOAT/1 -> Reset power 1/1(Power), Reset power 3/1(Power), Reset power 4/1(Power), Reset power 2/1(Power)
  Reset power 2/1(Error) -> OR/2
  Reset power 1/1(Error) -> OR/1
  Reset power 3/1(Error) -> OR/3
  Reset power 4/1(Error) -> OR/4
  OR/1 -> Error/1

== system BrickPi/Reset_all/Reset sensor ports ==
  OR : Logic  Operator=OR  Inputs=4  IconShape=distinctive  AllPortsSameDT=off  OutDataTypeStr=boolean
  Reset sensor port 1 : Subsystem
      mask Display: disp('Set sensor type')
  Reset sensor port 2 : Subsystem
      mask Display: disp('Set sensor type')
  Reset sensor port 3 : Subsystem
      mask Display: disp('Set sensor type')
  Reset sensor port 4 : Subsystem
      mask Display: disp('Set sensor type')
  Error : Outport
  wires:
  Reset sensor port 2/1(Error) -> OR/2
  Reset sensor port 3/1(Error) -> OR/3
  OR/1 -> Error/1
  Reset sensor port 1/1(Error) -> OR/1
  Reset sensor port 4/1(Error) -> OR/4

== system BrickPi/Touch/Get_sensor_value ==
  note: Get sensor value
  SensorPort : Inport
  SensorType : Inport  Port=2  OutDataTypeStr=uint8
  Enable : EnablePort
  0xA5 : Constant  Value=165
  "Address " : Constant  OutDataTypeStr=uint8
  Address3 : Constant  Value=[0 0 0 0 0]  OutDataTypeStr=uint8
  Bytes[3-6] : Selector  IndexMode=Zero-based  InputPortWidth=7  IndexOptions=Index vector (dialog)  Indices=[3 4 5 6]  OutputSizes=1
  Demux : Demux
  Equal : RelationalOperator  Operator=~=  OutDataTypeStr=boolean  RndMeth=Simplest
  Equal1 : RelationalOperator  Operator=~=  OutDataTypeStr=boolean  RndMeth=Simplest
  Equal2 : RelationalOperator  Operator=~=  OutDataTypeStr=boolean  RndMeth=Simplest
  Mux : Mux  Inputs=3
  Mux2 : Mux  Inputs=3
  SPI Master Transfer2 : raspberrypilib/SPI Master Transfer  Priority=6  BoardProperty=Pi 3 Model B  SPIModule=uint32(0)  Mode=Master  BusSpeed=1000000  Pin=SPI0_CE1  FirstBitToTransfer=Most significant bit (MSB)  ClockMode=0  BlockFunction=Transfer  RegisterAddress=0  OutputDataType=int8  OutputDataLength=1
      settings: SourceProductName=Simulink Support Package for Raspberry Pi Hardware  SourceProductBaseCode=RASPPI
  SPI_MSG_GET_ SENSOR offset : Constant  Value=12  OutMin=[1]  OutMax=[28]  OutDataTypeStr=uint8
  Sensor type offset : Constant  Value=4  OutDataTypeStr=uint8
  Sum : Sum  OutDataTypeStr=uint8
  Sum1 : Sum
  Valid data : Constant  Value=0  OutDataTypeStr=uint8
  Value : Outport
  Error : Outport  Port=2
  wires:
  Address3/1 -> Mux2/3
  SPI Master Transfer2/1 -> Bytes[3-6]/1
  Mux2/1 -> SPI Master Transfer2/1
  "Address "/1 -> Mux2/1
  Sum/1 -> Mux2/2
  SPI_MSG_GET_ SENSOR offset/1 -> Sum/2
  SensorPort/1 -> Sum/1
  Bytes[3-6]/1 -> Demux/1
  Demux/2 -> Equal/2
  Demux/4 -> Value/1
  0xA5/1 -> Equal2/1
  Valid data/1 -> Equal1/2
  Demux/3 -> Equal1/1
  Equal/1 -> Mux/2
  Mux/1 -> Error/1
  Equal1/1 -> Mux/3
  Demux/1 -> Equal2/2
  Equal2/1 -> Mux/1
  Sum1/1 -> Equal/1
  SensorType/1 -> Sum1/1
  Sensor type offset/1 -> Sum1/2

== system BrickPi/Touch/Set_sensor_type ==
  note: Check whether 4th element == 0xA5?
  note: Set sensor type
  SensorPort : Inport  OutDataTypeStr=uint8
  SensorType : Inport  Port=2  OutDataTypeStr=uint8
  Enable : EnablePort
  0xA5 : Constant  Value=165
  Address : Constant  VectorParams1D=off  OutDataTypeStr=uint8
  Constant2 : Constant  OutDataTypeStr=uint8
  Constant3 : Constant  OutDataTypeStr=uint8
  Mux1 : Mux
  NAND : Logic  Operator=NAND  IconShape=distinctive  AllPortsSameDT=off  OutDataTypeStr=boolean
  SPI Master Transfer1 : raspberrypilib/SPI Master Transfer  Priority=1  BoardProperty=Pi 3 Model B  SPIModule=uint32(0)  Mode=Master  BusSpeed=1000000  Pin=SPI0_CE1  FirstBitToTransfer=Most significant bit (MSB)  ClockMode=0  BlockFunction=Transfer  RegisterAddress=0  OutputDataType=int8  OutputDataLength=1
      settings: SourceProductName=Simulink Support Package for Raspberry Pi Hardware  SourceProductBaseCode=RASPPI
  SPI_MSG_SET_ SENSOR_TYPE : Constant  Value=12  OutMin=[1]  OutMax=[28]  OutDataTypeStr=uint8
  Selector1 : Selector  InputPortWidth=4  IndexOptions=Index vector (dialog)  Indices=[4]  OutputSizes=1
  Sensor type offset : Constant  Value=4  OutDataTypeStr=uint8
  Shift Arithmetic : ArithShift  BitShiftNumberSource=Input port  BitShiftNumber=8  BitShiftDirection=Left
      settings: InputPortMap=u0,p1
  Subtract : Sum  Inputs=+-
  Sum : Sum
  Error : Outport  InitialOutput=[1]
  wires:
  Mux1/1 -> SPI Master Transfer1/1
  SPI Master Transfer1/1 -> Selector1/1
  Address/1 -> Mux1/1
  SPI_MSG_SET_ SENSOR_TYPE/1 -> Mux1/2
  Selector1/1 -> NAND/1
  0xA5/1 -> NAND/2
  NAND/1 -> Error/1
  Subtract/1 -> Shift Arithmetic/2
  Constant3/1 -> Subtract/2
  SensorPort/1 -> Subtract/1
  Constant2/1 -> Shift Arithmetic/1
  Shift Arithmetic/1 -> Mux1/3
  Sum/1 -> Mux1/4
  SensorType/1 -> Sum/1
  Sensor type offset/1 -> Sum/2

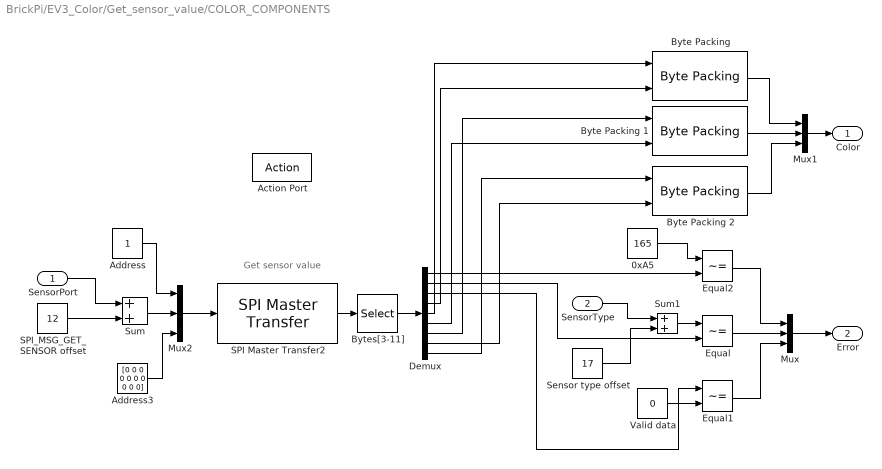
== system BrickPi/EV3_Color/Get_sensor_value/COLOR_COMPONENTS ==
  note: Get sensor value
  SensorPort : Inport
  SensorType : Inport  Port=2  OutDataTypeStr=uint8
  Action Port : ActionPort  ActionType=case
  0xA5 : Constant  Value=165
  "Address " : Constant  OutDataTypeStr=uint8
  Address3 : Constant  Value=[0 0 0 0 0 0 0 0 0 0]  OutDataTypeStr=uint8
  "Byte Packing " : xpcutilitieslib/Byte Packing   MaskPackedDataType=int16  MaskUnpackedDataTypes={'uint8', 'uint8'}  MaskAlignment=1
  Byte Packing 1 : xpcutilitieslib/Byte Packing   MaskPackedDataType=int16  MaskUnpackedDataTypes={'uint8', 'uint8'}  MaskAlignment=1
  Byte Packing 2 : xpcutilitieslib/Byte Packing   MaskPackedDataType=int16  MaskUnpackedDataTypes={'uint8', 'uint8'}  MaskAlignment=1
  Bytes[3-11] : Selector  IndexMode=Zero-based  InputPortWidth=12  IndexOptions=Index vector (dialog)  Indices=[3 4 5 6 7 8 9 10 11]  OutputSizes=1
  Demux : Demux  Outputs=9
  Equal : RelationalOperator  Operator=~=  OutDataTypeStr=boolean  RndMeth=Simplest
  Equal1 : RelationalOperator  Operator=~=  OutDataTypeStr=boolean  RndMeth=Simplest
  Equal2 : RelationalOperator  Operator=~=  OutDataTypeStr=boolean  RndMeth=Simplest
  Mux : Mux  Inputs=3
  Mux1 : Mux  Inputs=3
  Mux2 : Mux  Inputs=3
  SPI Master Transfer2 : raspberrypilib/SPI Master Transfer  Priority=6  BoardProperty=Pi 3 Model B  SPIModule=uint32(0)  Mode=Master  BusSpeed=1000000  Pin=SPI0_CE1  FirstBitToTransfer=Most significant bit (MSB)  ClockMode=0  BlockFunction=Transfer  RegisterAddress=0  OutputDataType=int8  OutputDataLength=1
      settings: SourceProductName=Simulink Support Package for Raspberry Pi Hardware  SourceProductBaseCode=RASPPI
  SPI_MSG_GET_ SENSOR offset : Constant  Value=12  OutMin=[1]  OutMax=[28]  OutDataTypeStr=uint8
  Sensor type offset : Constant  Value=17  OutDataTypeStr=uint8
  Sum : Sum  OutDataTypeStr=uint8
  Sum1 : Sum
  Valid data : Constant  Value=0  OutDataTypeStr=uint8
  Color : Outport
  Error : Outport  Port=2
  wires:
  Sum1/1 -> Equal/1
  0xA5/1 -> Equal2/1
  Equal2/1 -> Mux/1
  SPI_MSG_GET_ SENSOR offset/1 -> Sum/2
  Valid data/1 -> Equal1/2
  Address3/1 -> Mux2/3
  Equal1/1 -> Mux/3
  Bytes[3-11]/1 -> Demux/1
  Demux/1 -> Equal2/2
  Mux2/1 -> SPI Master Transfer2/1
  Demux/2 -> Equal/2
  SensorPort/1 -> Sum/1
  Sensor type offset/1 -> Sum1/2
  Equal/1 -> Mux/2
  Mux/1 -> Error/1
  Sum/1 -> Mux2/2
  SPI Master Transfer2/1 -> Bytes[3-11]/1
  SensorType/1 -> Sum1/1
  "Address "/1 -> Mux2/1
  Demux/3 -> Equal1/1
  Mux1/1 -> Color/1
  "Byte Packing "/1 -> Mux1/1
  Byte Packing 1/1 -> Mux1/2
  Byte Packing 2/1 -> Mux1/3
  Demux/4 -> "Byte Packing "/2
  Demux/5 -> "Byte Packing "/1
  Demux/7 -> Byte Packing 1/1
  Demux/6 -> Byte Packing 1/2
  Demux/8 -> Byte Packing 2/2
  Demux/9 -> Byte Packing 2/1

== system BrickPi/EV3_Color/Get_sensor_value/COLOR_RAW_REFLECTED ==
  note: Get sensor value
  SensorPort : Inport
  SensorType : Inport  Port=2  OutDataTypeStr=uint8
  Action Port : ActionPort  ActionType=case
  0xA5 : Constant  Value=165
  "Address " : Constant  OutDataTypeStr=uint8
  Address3 : Constant  Value=[0 0 0 0 0 0]  OutDataTypeStr=uint8
  "Byte Packing " : xpcutilitieslib/Byte Packing   MaskPackedDataType=int16  MaskUnpackedDataTypes={'uint8', 'uint8'}  MaskAlignment=1
  Bytes[3-7] : Selector  IndexMode=Zero-based  InputPortWidth=8  IndexOptions=Index vector (dialog)  Indices=[3 4 5 6 7]  OutputSizes=1
  Demux : Demux  Outputs=5
  Equal : RelationalOperator  Operator=~=  OutDataTypeStr=boolean  RndMeth=Simplest
  Equal1 : RelationalOperator  Operator=~=  OutDataTypeStr=boolean  RndMeth=Simplest
  Equal2 : RelationalOperator  Operator=~=  OutDataTypeStr=boolean  RndMeth=Simplest
  Mux : Mux  Inputs=3
  Mux2 : Mux  Inputs=3
  SPI Master Transfer2 : raspberrypilib/SPI Master Transfer  Priority=6  BoardProperty=Pi 3 Model B  SPIModule=uint32(0)  Mode=Master  BusSpeed=1000000  Pin=SPI0_CE1  FirstBitToTransfer=Most significant bit (MSB)  ClockMode=0  BlockFunction=Transfer  RegisterAddress=0  OutputDataType=int8  OutputDataLength=1
      settings: SourceProductName=Simulink Support Package for Raspberry Pi Hardware  SourceProductBaseCode=RASPPI
  SPI_MSG_GET_ SENSOR offset : Constant  Value=12  OutMin=[1]  OutMax=[28]  OutDataTypeStr=uint8
  Sensor type offset : Constant  Value=17  OutDataTypeStr=uint8
  Sum : Sum  OutDataTypeStr=uint8
  Sum1 : Sum
  Valid data : Constant  Value=0  OutDataTypeStr=uint8
  Raw_red : Outport
  Error : Outport  Port=2
  wires:
  Sum1/1 -> Equal/1
  0xA5/1 -> Equal2/1
  Equal2/1 -> Mux/1
  SPI_MSG_GET_ SENSOR offset/1 -> Sum/2
  Valid data/1 -> Equal1/2
  Address3/1 -> Mux2/3
  Equal1/1 -> Mux/3
  Bytes[3-7]/1 -> Demux/1
  Demux/1 -> Equal2/2
  Mux2/1 -> SPI Master Transfer2/1
  Demux/2 -> Equal/2
  SensorPort/1 -> Sum/1
  Sensor type offset/1 -> Sum1/2
  Equal/1 -> Mux/2
  Mux/1 -> Error/1
  Sum/1 -> Mux2/2
  SPI Master Transfer2/1 -> Bytes[3-7]/1
  SensorType/1 -> Sum1/1
  "Address "/1 -> Mux2/1
  Demux/3 -> Equal1/1
  "Byte Packing "/1 -> Raw_red/1
  Demux/4 -> "Byte Packing "/2
  Demux/5 -> "Byte Packing "/1

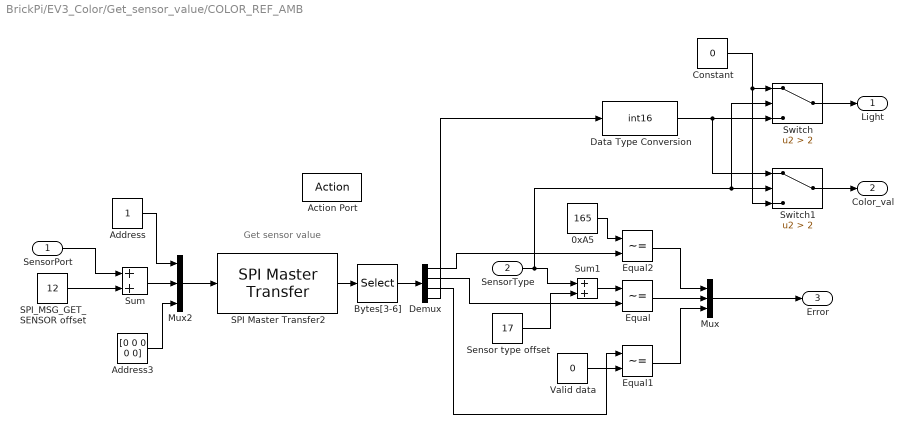
== system BrickPi/EV3_Color/Get_sensor_value/COLOR_REF_AMB ==
  note: Get sensor value
  SensorPort : Inport
  SensorType : Inport  Port=2  OutDataTypeStr=uint8
  Action Port : ActionPort  ActionType=case
  0xA5 : Constant  Value=165
  "Address " : Constant  OutDataTypeStr=uint8
  Address3 : Constant  Value=[0 0 0 0 0]  OutDataTypeStr=uint8
  Bytes[3-6] : Selector  IndexMode=Zero-based  InputPortWidth=7  IndexOptions=Index vector (dialog)  Indices=[3 4 5 6]  OutputSizes=1
  Constant : Constant  Value=0
  Data Type Conversion : DataTypeConversion  OutDataTypeStr=int16
  Demux : Demux
  Equal : RelationalOperator  Operator=~=  OutDataTypeStr=boolean  RndMeth=Simplest
  Equal1 : RelationalOperator  Operator=~=  OutDataTypeStr=boolean  RndMeth=Simplest
  Equal2 : RelationalOperator  Operator=~=  OutDataTypeStr=boolean  RndMeth=Simplest
  Mux : Mux  Inputs=3
  Mux2 : Mux  Inputs=3
  SPI Master Transfer2 : raspberrypilib/SPI Master Transfer  Priority=6  BoardProperty=Pi 3 Model B  SPIModule=uint32(0)  Mode=Master  BusSpeed=1000000  Pin=SPI0_CE1  FirstBitToTransfer=Most significant bit (MSB)  ClockMode=0  BlockFunction=Transfer  RegisterAddress=0  OutputDataType=int8  OutputDataLength=1
      settings: SourceProductName=Simulink Support Package for Raspberry Pi Hardware  SourceProductBaseCode=RASPPI
  SPI_MSG_GET_ SENSOR offset : Constant  Value=12  OutMin=[1]  OutMax=[28]  OutDataTypeStr=uint8
  Sensor type offset : Constant  Value=17  OutDataTypeStr=uint8
  Sum : Sum  OutDataTypeStr=uint8
  Sum1 : Sum
  Switch : Switch  Criteria=u2 > Threshold  Threshold=2
  Switch1 : Switch  Criteria=u2 > Threshold  Threshold=2
  Valid data : Constant  Value=0  OutDataTypeStr=uint8
  Light : Outport
  Color_val : Outport  Port=2
  Error : Outport  Port=3
  wires:
  Sum1/1 -> Equal/1
  0xA5/1 -> Equal2/1
  Equal2/1 -> Mux/1
  SPI_MSG_GET_ SENSOR offset/1 -> Sum/2
  Valid data/1 -> Equal1/2
  Address3/1 -> Mux2/3
  Equal1/1 -> Mux/3
  Bytes[3-6]/1 -> Demux/1
  Demux/1 -> Equal2/2
  Mux2/1 -> SPI Master Transfer2/1
  Demux/2 -> Equal/2
  SensorPort/1 -> Sum/1
  Sensor type offset/1 -> Sum1/2
  Equal/1 -> Mux/2
  Mux/1 -> Error/1
  Sum/1 -> Mux2/2
  SPI Master Transfer2/1 -> Bytes[3-6]/1
  SensorType/1 -> Switch/2, Switch1/2, Sum1/1
  Demux/4 -> Data Type Conversion/1
  "Address "/1 -> Mux2/1
  Demux/3 -> Equal1/1
  Switch/1 -> Light/1
  Switch1/1 -> Color_val/1
  Data Type Conversion/1 -> Switch1/1, Switch/3
  Constant/1 -> Switch/1, Switch1/3

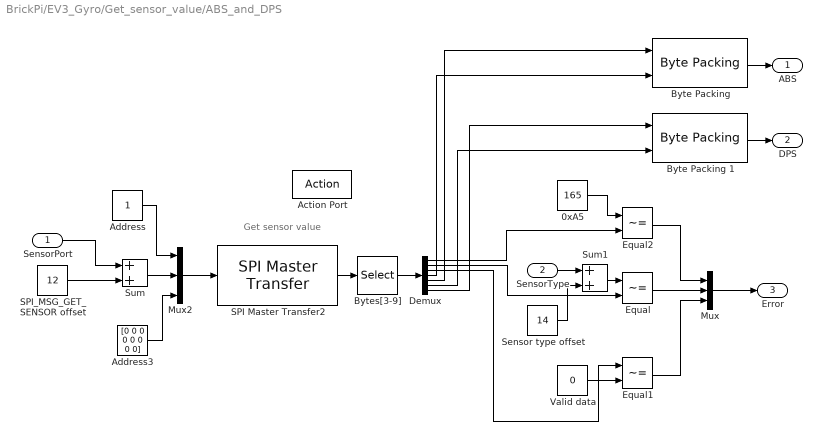
== system BrickPi/EV3_Gyro/Get_sensor_value/ABS_and_DPS ==
  note: Get sensor value
  SensorPort : Inport
  SensorType : Inport  Port=2  OutDataTypeStr=uint8
  Action Port : ActionPort
  0xA5 : Constant  Value=165
  "Address " : Constant  OutDataTypeStr=uint8
  Address3 : Constant  Value=[0 0 0 0 0 0 0 0]  OutDataTypeStr=uint8
  "Byte Packing " : xpcutilitieslib/Byte Packing   MaskPackedDataType=int16  MaskUnpackedDataTypes={'uint8', 'uint8'}  MaskAlignment=1
  Byte Packing 1 : xpcutilitieslib/Byte Packing   MaskPackedDataType=int16  MaskUnpackedDataTypes={'uint8', 'uint8'}  MaskAlignment=1
  Bytes[3-9] : Selector  IndexMode=Zero-based  InputPortWidth=10  IndexOptions=Index vector (dialog)  Indices=[3 4 5 6 7 8 9]  OutputSizes=1
  Demux : Demux  Outputs=7
  Equal : RelationalOperator  Operator=~=  OutDataTypeStr=boolean  RndMeth=Simplest
  Equal1 : RelationalOperator  Operator=~=  OutDataTypeStr=boolean  RndMeth=Simplest
  Equal2 : RelationalOperator  Operator=~=  OutDataTypeStr=boolean  RndMeth=Simplest
  Mux : Mux  Inputs=3
  Mux2 : Mux  Inputs=3
  SPI Master Transfer2 : raspberrypilib/SPI Master Transfer  Priority=6  BoardProperty=Pi 3 Model B  SPIModule=uint32(0)  Mode=Master  BusSpeed=1000000  Pin=SPI0_CE1  FirstBitToTransfer=Most significant bit (MSB)  ClockMode=0  BlockFunction=Transfer  RegisterAddress=0  OutputDataType=int8  OutputDataLength=1
      settings: SourceProductName=Simulink Support Package for Raspberry Pi Hardware  SourceProductBaseCode=RASPPI
  SPI_MSG_GET_ SENSOR offset : Constant  Value=12  OutMin=[1]  OutMax=[28]  OutDataTypeStr=uint8
  Sensor type offset : Constant  Value=14  OutDataTypeStr=uint8
  Sum : Sum  OutDataTypeStr=uint8
  Sum1 : Sum  OutDataTypeStr=uint8
  Valid data : Constant  Value=0  OutDataTypeStr=uint8
  ABS : Outport
  DPS : Outport  Port=2
  Error : Outport  Port=3
  wires:
  SPI_MSG_GET_ SENSOR offset/1 -> Sum/2
  Equal2/1 -> Mux/1
  Address3/1 -> Mux2/3
  Mux2/1 -> SPI Master Transfer2/1
  Mux/1 -> Error/1
  Bytes[3-9]/1 -> Demux/1
  Equal1/1 -> Mux/3
  Demux/3 -> Equal1/1
  SensorPort/1 -> Sum/1
  Demux/1 -> Equal2/2
  "Address "/1 -> Mux2/1
  Valid data/1 -> Equal1/2
  0xA5/1 -> Equal2/1
  Equal/1 -> Mux/2
  Demux/2 -> Equal/2
  SPI Master Transfer2/1 -> Bytes[3-9]/1
  Sum/1 -> Mux2/2
  "Byte Packing "/1 -> ABS/1
  Byte Packing 1/1 -> DPS/1
  Sum1/1 -> Equal/1
  SensorType/1 -> Sum1/1
  Sensor type offset/1 -> Sum1/2
  Demux/5 -> "Byte Packing "/1
  Demux/4 -> "Byte Packing "/2
  Demux/7 -> Byte Packing 1/1
  Demux/6 -> Byte Packing 1/2

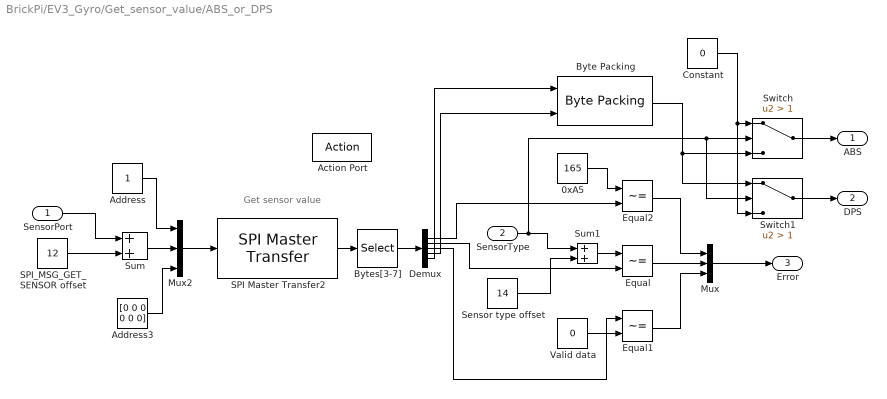
== system BrickPi/EV3_Gyro/Get_sensor_value/ABS_or_DPS ==
  note: Get sensor value
  SensorPort : Inport
  SensorType : Inport  Port=2  OutDataTypeStr=uint8
  Action Port : ActionPort
  0xA5 : Constant  Value=165
  "Address " : Constant  OutDataTypeStr=uint8
  Address3 : Constant  Value=[0 0 0 0 0 0]  OutDataTypeStr=uint8
  "Byte Packing " : xpcutilitieslib/Byte Packing   MaskPackedDataType=int16  MaskUnpackedDataTypes={'uint8', 'uint8'}  MaskAlignment=1
  Bytes[3-7] : Selector  IndexMode=Zero-based  InputPortWidth=8  IndexOptions=Index vector (dialog)  Indices=[3 4 5 6 7]  OutputSizes=1
  Constant : Constant  Value=0  OutDataTypeStr=uint8
  Demux : Demux  Outputs=5
  Equal : RelationalOperator  Operator=~=  OutDataTypeStr=boolean  RndMeth=Simplest
  Equal1 : RelationalOperator  Operator=~=  OutDataTypeStr=boolean  RndMeth=Simplest
  Equal2 : RelationalOperator  Operator=~=  OutDataTypeStr=boolean  RndMeth=Simplest
  Mux : Mux  Inputs=3
  Mux2 : Mux  Inputs=3
  SPI Master Transfer2 : raspberrypilib/SPI Master Transfer  Priority=6  BoardProperty=Pi 3 Model B  SPIModule=uint32(0)  Mode=Master  BusSpeed=1000000  Pin=SPI0_CE1  FirstBitToTransfer=Most significant bit (MSB)  ClockMode=0  BlockFunction=Transfer  RegisterAddress=0  OutputDataType=int8  OutputDataLength=1
      settings: SourceProductName=Simulink Support Package for Raspberry Pi Hardware  SourceProductBaseCode=RASPPI
  SPI_MSG_GET_ SENSOR offset : Constant  Value=12  OutMin=[1]  OutMax=[28]  OutDataTypeStr=uint8
  Sensor type offset : Constant  Value=14  OutDataTypeStr=uint8
  Sum : Sum  OutDataTypeStr=uint8
  Sum1 : Sum
  Switch : Switch  Criteria=u2 > Threshold  Threshold=1
  Switch1 : Switch  Criteria=u2 > Threshold  Threshold=1
  Valid data : Constant  Value=0  OutDataTypeStr=uint8
  ABS : Outport
  DPS : Outport  Port=2
  Error : Outport  Port=3
  wires:
  SensorType/1 -> Switch1/2, Switch/2, Sum1/1
  Sensor type offset/1 -> Sum1/2
  SPI_MSG_GET_ SENSOR offset/1 -> Sum/2
  Equal2/1 -> Mux/1
  Address3/1 -> Mux2/3
  Mux2/1 -> SPI Master Transfer2/1
  Mux/1 -> Error/1
  Bytes[3-7]/1 -> Demux/1
  Equal1/1 -> Mux/3
  Demux/3 -> Equal1/1
  SensorPort/1 -> Sum/1
  Demux/1 -> Equal2/2
  Sum1/1 -> Equal/1
  "Address "/1 -> Mux2/1
  Valid data/1 -> Equal1/2
  0xA5/1 -> Equal2/1
  Equal/1 -> Mux/2
  Demux/2 -> Equal/2
  SPI Master Transfer2/1 -> Bytes[3-7]/1
  Sum/1 -> Mux2/2
  Constant/1 -> Switch1/3, Switch/1
  Switch1/1 -> DPS/1
  Switch/1 -> ABS/1
  "Byte Packing "/1 -> Switch/3, Switch1/1
  Demux/4 -> "Byte Packing "/2
  Demux/5 -> "Byte Packing "/1

== system BrickPi/EV3_Infrared/Get_sensor_value/Subsystem ==
  note: Get sensor value
  SensorPort : Inport
  SensorType : Inport  Port=2  OutDataTypeStr=uint8
  Action Port : ActionPort  ActionType=case
  0xA5 : Constant  Value=165
  "Address " : Constant  OutDataTypeStr=uint8
  Address3 : Constant  Value=[0 0 0 0 0]  OutDataTypeStr=uint8
  Bytes[3-6] : Selector  IndexMode=Zero-based  InputPortWidth=7  IndexOptions=Index vector (dialog)  Indices=[3 4 5 6]  OutputSizes=1
  Demux : Demux
  Equal : RelationalOperator  Operator=~=  OutDataTypeStr=boolean  RndMeth=Simplest
  Equal1 : RelationalOperator  Operator=~=  OutDataTypeStr=boolean  RndMeth=Simplest
  Equal2 : RelationalOperator  Operator=~=  OutDataTypeStr=boolean  RndMeth=Simplest
  Mux : Mux  Inputs=3
  Mux2 : Mux  Inputs=3
  SPI Master Transfer2 : raspberrypilib/SPI Master Transfer  Priority=6  BoardProperty=Pi 3 Model B  SPIModule=uint32(0)  Mode=Master  BusSpeed=1000000  Pin=SPI0_CE1  FirstBitToTransfer=Most significant bit (MSB)  ClockMode=0  BlockFunction=Transfer  RegisterAddress=0  OutputDataType=int8  OutputDataLength=1
      settings: SourceProductName=Simulink Support Package for Raspberry Pi Hardware  SourceProductBaseCode=RASPPI
  SPI_MSG_GET_ SENSOR offset : Constant  Value=12  OutMin=[1]  OutMax=[28]  OutDataTypeStr=uint8
  Sum : Sum  OutDataTypeStr=uint8
  Sum1 : Sum  OutDataTypeStr=uint8
  Type Offset : Constant  Value=25  OutDataTypeStr=uint8
  Valid data : Constant  Value=0  OutDataTypeStr=uint8
  Proximity : Outport
  Error : Outport  Port=2
  wires:
  Equal2/1 -> Mux/1
  Demux/1 -> Equal2/2
  SPI_MSG_GET_ SENSOR offset/1 -> Sum/2
  Demux/3 -> Equal1/1
  Equal/1 -> Mux/2
  Demux/4 -> Proximity/1
  Demux/2 -> Equal/2
  Equal1/1 -> Mux/3
  "Address "/1 -> Mux2/1
  Valid data/1 -> Equal1/2
  Mux/1 -> Error/1
  Mux2/1 -> SPI Master Transfer2/1
  SPI Master Transfer2/1 -> Bytes[3-6]/1
  Bytes[3-6]/1 -> Demux/1
  Address3/1 -> Mux2/3
  SensorPort/1 -> Sum/1
  Sum/1 -> Mux2/2
  0xA5/1 -> Equal2/1
  Sum1/1 -> Equal/1
  SensorType/1 -> Sum1/1
  Type Offset/1 -> Sum1/2
